simulink model "Simulation_model_of_fuzzy_shift_control_system"  (R2014b)
settings: Solver=ode45  StartTime=0.0  StopTime=20  RelTol=1e-3
undefined symbols (not defined in the file): sigbuilder_block
libraries: fuzblock x1
settings Model: Creator=Administrator  LastModifiedBy=gd

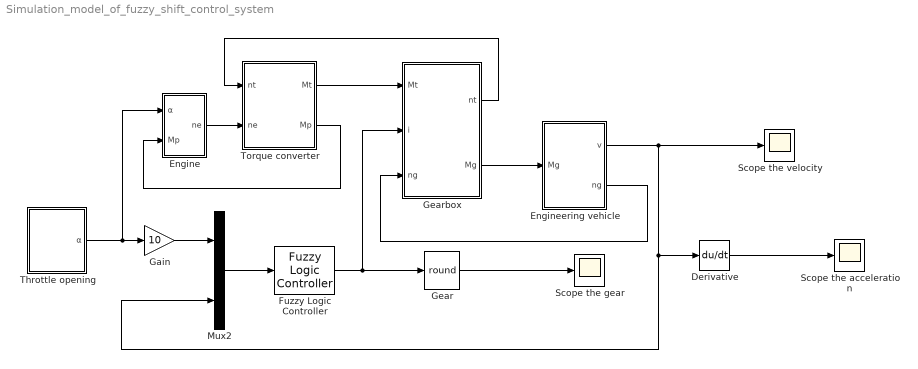
== system Simulation_model_of_fuzzy_shift_control_system ==
  Derivative : Derivative
  Engine : Subsystem
  Engineering vehicle : Subsystem
  Fuzzy Logic Controller : fuzblock/Fuzzy Logic  Controller  fis=Fuzzy_logic_control_rules
  Gain : Gain  Gain=10
  Gear : Rounding  Operator=round
  Gearbox : Subsystem
  Mux2 : Mux  Inputs=2
  Scope the acceleration : Scope
      settings: TimeRange=150  YMin=1.2625  YMax=1.2975  SaveName=v2
  Scope the gear : Scope
      settings: YMin=1  YMax=4
  Scope the velocity : Scope
      settings: TimeRange=11  YMin=7  YMax=8.8  SaveName=v3
  Throttle opening : Subsystem  Tag=STV Subsys  LoadFcn=sigbuilder_block('load');  StartFcn=sigbuilder_block('start');  StopFcn=sigbuilder_block('stop');  ClipboardFcn=sigbuilder_block('clipboard');  mask(Sigbuilder block){}
      mask help: Simulink:masks:SigbuilderBlock_MD
      mask init:
      | if ~strcmp(get_param(bdroot(gcbh),'SimulationStatus'),'stopped') tuvar = sigbuilder_block('maskInit'); end
      settings: CopyFcn=sigbuilder_block('copy');  DeleteFcn=sigbuilder_block('delete');  ModelCloseFcn=sigbuilder_block('modelClose');  PreSaveFcn=sigbuilder_block('preSave');  PauseFcn=sigbuilder_block('pause');  ContinueFcn=sigbuilder_block('continue');  NameChangeFcn=sigbuilder_block('namechange');  OpenFcn=sigbuilder_block('open',[437.6 199.2 550.4 400 ]);  CloseFcn=sigbuilder_block('close');
      mask Display: plot(0, 0, 100, 100,[2, 2, 32, 32, 2], [68, 8, 8, 68, 68],[32, 2], [38, 38], [32, 19, 2],[53, 60, 44], [32, 17, 17, 2],[16, 16, 31, 31]);txt = getActiveGroup(gcbh);text(2, 100, txt,'verticalAlignment', 'top');
  Torque converter : Subsystem
  wires:
  Engine/1(ne) -> Torque converter/2(ne)
  Torque converter/1(Mt) -> Gearbox/1(Mt)
  Gearbox/1(nt) -> Torque converter/1(nt)
  Throttle opening/1(α) -> Engine/1(α), Gain/1
  Engineering vehicle/2(ng) -> Gearbox/3(ng)
  Torque converter/2(Mp) -> Engine/2(Mp)
  Fuzzy Logic Controller/1 -> Gearbox/2(i), Gear/1
  Gearbox/2(Mg) -> Engineering vehicle/1(Mg)
  Gear/1 -> Scope the gear/1
  Derivative/1 -> Scope the acceleration/1
  Gain/1 -> Mux2/1
  Engineering vehicle/1(v) -> Mux2/2, Derivative/1, Scope the velocity/1
  Mux2/1 -> Fuzzy Logic Controller/1

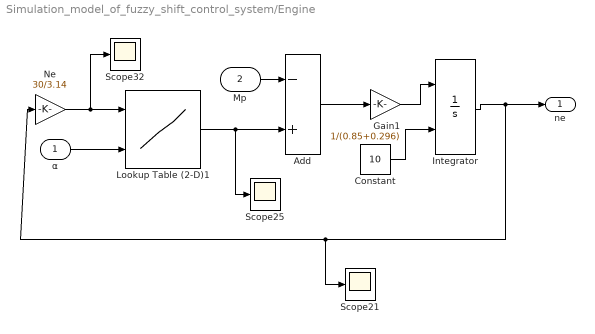
== system Simulation_model_of_fuzzy_shift_control_system/Engine ==
  α : Inport
  Mp : Inport  Port=2
  Add : Sum  Inputs=-+
  Constant : Constant  Value=10
  Gain1 : Gain  Gain=1/(0.85+0.296)
  Integrator : Integrator  InitialConditionSource=external  InitialCondition=150  LimitOutput=on  UpperSaturationLimit=2400*2*3.14/60  LowerSaturationLimit=800*2*3.14/60
  Lookup Table (2-D)1 : Lookup2D  RowIndex=[800,900,1000,1120,1200,1300,1410,1510,1620,1720,1807,1900,2030,2130,2230,2400]  ColumnIndex=[0.4,0.5,0.6,0.7,0.8,0.9,1]  Table=reshape([351,0,0,0,0,0,0,0,0,0,0,0,0,0,0,0,351,694,1380,0,0,0,0,0,0,0,0,0,0,0,0,0,351,694,1380,2067,2363,0,0,0,0,0,0,0,0,0,0,0,351,694,1380,2067,2363,2656.5,2529,0,0,0,0,0,0,0,0,0,351,694,1380,2067,2363,2656.5,2529,2465,2362,0,0,0,0,0,0,0,351,694,1380,2067,2363,2656.5,2529,2465,2362,2256,2146,0,0,0,0,0,351,694,1380,2067,2363,2656.5,2529,2465,2362,2256,2146,2073,1953,1862,1761,1662],16,7)
  Ne : Gain  Gain=30/3.14
  Scope21 : Scope
      settings: YMin=3.8  YMax=4.2  SaveName=ScopeData4
  Scope25 : Scope
      settings: YMin=3.8  YMax=4.2  SaveName=ScopeData3
  Scope32 : Scope
      settings: YMin=3.8  YMax=4.2  SaveName=ScopeData10
  ne : Outport
  wires:
  Lookup Table (2-D)1/1 -> Scope25/1, Add/2
  Add/1 -> Gain1/1
  Gain1/1 -> Integrator/1
  Integrator/1 -> ne/1, Ne/1, Scope21/1
  Mp/1 -> Add/1
  Constant/1 -> Integrator/2
  Ne/1 -> Lookup Table (2-D)1/1, Scope32/1
  α/1 -> Lookup Table (2-D)1/2

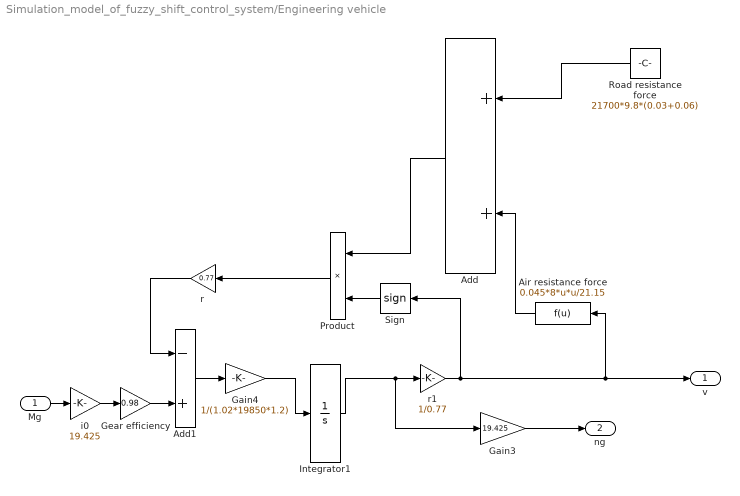
== system Simulation_model_of_fuzzy_shift_control_system/Engineering vehicle ==
  Mg : Inport
  Add : Sum
  Add1 : Sum  Inputs=-+
  Air resistance force : Fcn  Expr=0.045*8*u*u/21.15
  Gain3 : Gain  Gain=19.425
  Gain4 : Gain  Gain=1/(1.02*19850*1.2)
  Gear efficiency : Gain  Gain=0.98
  Integrator1 : Integrator  UpperSaturationLimit=20  LowerSaturationLimit=-20
  Product : Product  RndMeth=Zero
  Road resistance force : Constant  Value=21700*9.8*(0.03+0.06)
  Sign : Signum
  i0 : Gain  Gain=19.425
  r : Gain  Gain=0.77
  r1 : Gain  Gain=1/0.77
  v : Outport
  ng : Outport  Port=2
  wires:
  Integrator1/1 -> r1/1, Gain3/1
  Gain3/1 -> ng/1
  Add/1 -> Product/1
  Air resistance force/1 -> Add/2
  i0/1 -> Gear efficiency/1
  Add1/1 -> Gain4/1
  Gain4/1 -> Integrator1/1
  Mg/1 -> i0/1
  Product/1 -> r/1
  r/1 -> Add1/1
  r1/1 -> Sign/1, v/1, Air resistance force/1
  Gear efficiency/1 -> Add1/2
  Sign/1 -> Product/2
  Road resistance force/1 -> Add/1

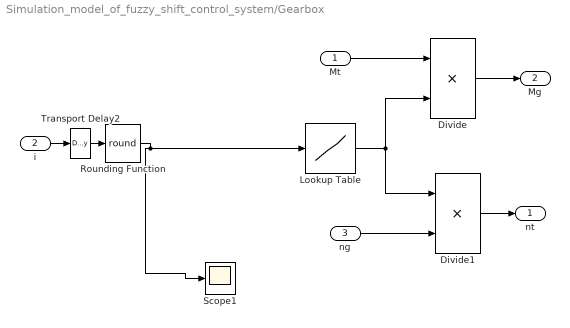
== system Simulation_model_of_fuzzy_shift_control_system/Gearbox ==
  Mt : Inport
  i : Inport  Port=2
  ng : Inport  Port=3
  Divide : Product  Inputs=**
  Divide1 : Product  Inputs=**
  Lookup Table : Lookup  InputValues=[1,2,3,4,5,6,7]  Table=[7.63 3.51 1.91 1.43 1 0.74 0.64]
  Rounding Function : Rounding  Operator=round
  Scope1 : Scope
      settings: YMin=1  YMax=2  SaveName=d1
  Transport Delay2 : TransportDelay  DelayTime=0.1
  nt : Outport
  Mg : Outport  Port=2
  wires:
  Lookup Table/1 -> Divide/2, Divide1/1
  Mt/1 -> Divide/1
  Divide1/1 -> nt/1
  Divide/1 -> Mg/1
  i/1 -> Transport Delay2/1
  ng/1 -> Divide1/2
  Rounding Function/1 -> Scope1/1, Lookup Table/1
  Transport Delay2/1 -> Rounding Function/1

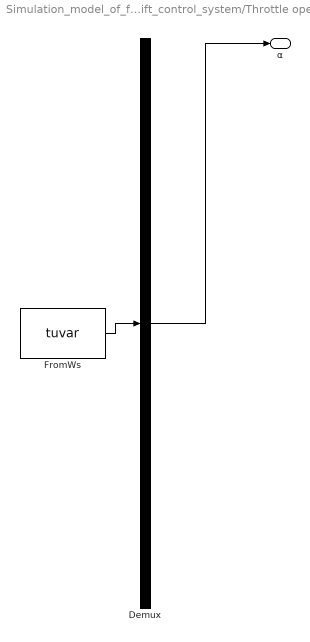
== system Simulation_model_of_fuzzy_shift_control_system/Throttle opening ==
  Demux : Demux  Tag=STV Demux  Outputs=1
  FromWs : FromWorkspace  Tag=STV FromWs  VariableName=tuvar  SampleTime=0
      SigBuilderData=|
      | common.afterFinalStr = 'Extrapolate'
      | common.sampleTime = 0
      | dataSet.timeRange = [0 10]
      | dataSet.name = 'Sheet'
      | sbobj.Name = 'Signal Builder'
      | sbobj.Groups.Name = 'Sheet'
      | sbobj.Groups.Signals.Name = 'α'
      | sbobj.Groups.Signals.XData = [0 1.25 2.5 3.75 5 6.25 7.5 8.75 10]
      | sbobj.Groups.Signals.YData = [0.2 0.3 0.4 0.5 0.6 0.7 0.8 0.9 1]
  α : Outport
  wires:
  Demux/1 -> α/1
  FromWs/1 -> Demux/1

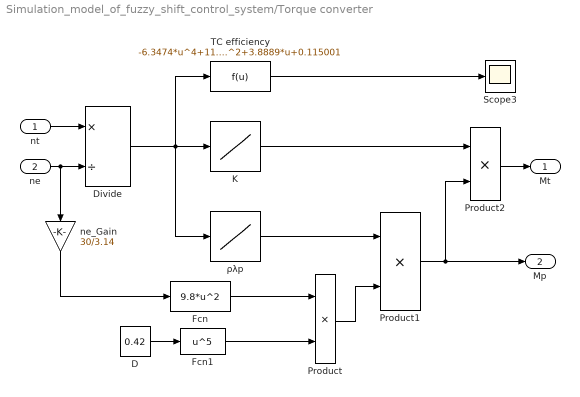
== system Simulation_model_of_fuzzy_shift_control_system/Torque converter ==
  nt : Inport
  ne : Inport  Port=2
  D : Constant  Value=0.42
  Divide : Product  Inputs=*/
  Fcn : Fcn  Expr=9.8*u^2
  Fcn1 : Fcn  Expr=u^5
  K : Lookup  InputValues=[0,0.06,0.1,0.15,0.2,0.24,0.3,0.43,0.51,0.56,0.6,0.64,0.7,0.77,0.82,0.86,0.88,0.92,0.99]  Table=[2.24,2.17,2.14,2.03,1.99,1.93,1.82,1.62,1.52,1.43,1.38,1.31,1.24,1.13,1.11,1.05,0.99,0.72,0.31]  LUTDesignUseExistingBP=off  LUTDesignAbsError=NaN
  Product : Product  RndMeth=Zero
  Product1 : Product  RndMeth=Zero
  Product2 : Product  RndMeth=Zero
  Scope3 : Scope
      settings: TimeRange=11  YMin=-0.1  YMax=0.9  SaveName=x1
  TC efficiency : Fcn  Expr=-6.3474*u^4+11.5425*u^3-8.7174*u^2+3.8889*u+0.115001
  ne_Gain : Gain  Gain=30/3.14
  ρλp : Lookup  InputValues=[0,0.06,0.1,0.15,0.2,0.24,0.3,0.43,0.51,0.56,0.6,0.64,0.7,0.77,0.82,0.86,0.88,0.92,0.99]  Table=[0.00149,0.00159,0.0016,0.00159,0.00157,0.00156,0.00155,0.00154,0.001536,0.00153,0.001525,0.00152,0.00149,0.00144,0.00137,0.00125,0.00115,0.00107,0.00082]  LUTDesignUseExistingBP=off  LUTDesignAbsError=NaN
  Mt : Outport
  Mp : Outport  Port=2
  wires:
  Divide/1 -> ρλp/1, K/1, TC efficiency/1
  ρλp/1 -> Product1/1
  D/1 -> Fcn1/1
  Fcn1/1 -> Product/2
  Product/1 -> Product1/2
  Product1/1 -> Product2/2, Mp/1
  K/1 -> Product2/1
  nt/1 -> Divide/1
  Product2/1 -> Mt/1
  ne_Gain/1 -> Fcn/1
  Fcn/1 -> Product/1
  TC efficiency/1 -> Scope3/1
  ne/1 -> Divide/2, ne_Gain/1
